simulink model "Lista3"  (R2023a)
settings: Solver=VariableStepAuto  StartTime=0.0  StopTime=10.0  RelTol=1e-3
libraries: fl_lib x5, nesl_utility x2
settings Model: Creator=gutoc  LastModifiedBy=gutoc

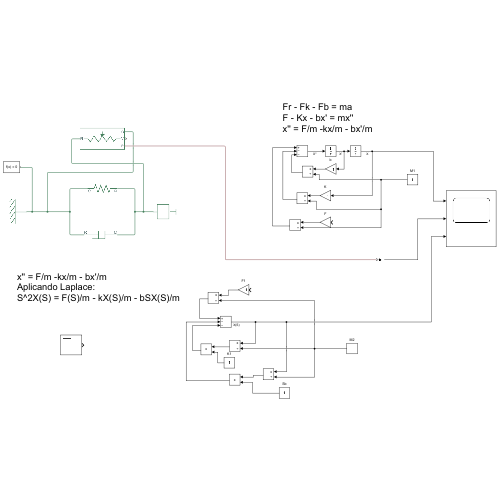
[thumbnail: Simulink's stored preview of the top-level diagram]
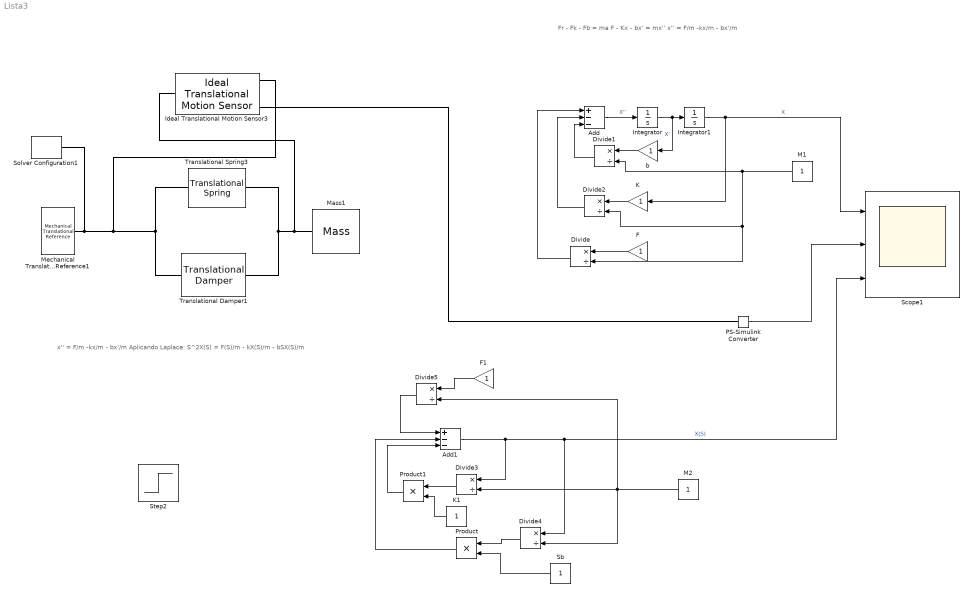
== system Lista3 ==
  note: x'' = F/m -kx/m - bx'/m
      | Aplicando Laplace:
      | S^2X(S) = F(S)/m - kX(S)/m - bSX(S)/m
  note: Fr - Fk - Fb = ma
      | F - Kx - bx' = mx''
      | x'' = F/m -kx/m - bx'/m
  Add : Sum  Inputs=+--
  Add1 : Sum  Inputs=+--
  Divide{,1..5} (6 alike) : Product  Inputs=*/
  F : Gain
  F1 : Gain
  Ideal Translational Motion Sensor3 : fl_lib/Mechanical/Mechanical Sensors/Ideal Translational Motion Sensor  reference=foundation.enum.MeasurementReference.difference  acceleration_port=false  velocity_port=true  position_port=true  offset=0 m
  Integrator : Integrator
  Integrator1 : Integrator
  K : Gain
  K1 : Constant
  M1 : Constant  VectorParams1D=off
  M2 : Constant  VectorParams1D=off
  Mass1 : fl_lib/Mechanical/Translational Elements/Mass  mass=10 kg  num_ports=foundation.enum.numPorts2.one  v_specify=on  v_priority=High  v=5 m/s  v_nominal_specify=off  v_nominal_unit=m/s  v_nominal_value=1  f_specify=off  f_priority=None  f=0 N  f_nominal_specify=off  f_nominal_unit=N  f_nominal_value=1
  Mechanical Translational Reference1 : fl_lib/Mechanical/Translational Elements/Mechanical Translational Reference
  PS-Simulink Converter : nesl_utility/PS-Simulink Converter  PhysicalDomain=network_engine_domain  SubClassName=ps_output  LeftPortType=input  RightPortType=output  PseudoPeriodic=off  Frequencies=[]  VectorFormat=inherit  Unit=inherit  AffineConversion=off
  Product : Product
  Product1 : Product
  Sb : Constant  VectorParams1D=off
  Scope1 : Scope  NumInputPorts=3
  Solver Configuration1 : nesl_utility/Solver Configuration  PhysicalDomain=network_engine_domain  SubClassName=solver  LeftPortType=input  RightPortType=generic  Tones=[]  Harmonics=[]  SimulateNoise=off  Profile=off  UseLocalSampling=off  EnableSwitchedLinearOptims=on  FrequencyDomain=off  UseCCode=off  RelTol=0.001  AbsTol=1e-06  MinStep=1e-09  ToWorkspace=off  RevertToSquareIcSolve=off  NumHomotopyIterations=100  PhasorMode=off  PhasorModeNumHarmonics=1  ConsistencySolver=NEWTON_FTOL  IndexReductionMethod=DerivativeReplacement  DoDC=off  ResidualTolerance=1e-09  ConsistencyTolSource=GLOBAL  ConsistencyAbsTol=0.001  ConsistencyRelTol=0.001  ConsistencyTolFactor=0.001  UseLocalSolver=off  LocalSolverChoice=NE_BACKWARD_EULER_ADVANCER  ResolveIndetEquations=on  FunctionEvalNumThread=1  LocalSolverSampleTime=0.001  DoFixedCost=off  MaxNonlinIter=3  MaxModeIter=2  ComputeImpulses=off  ImpulseIterations=2  LinearAlgebra=Sparse  LinearAlgebraNumThread=0  EquationFormulation=NE_TIME_EF  DelaysMemoryBudget=1024  AutomaticFiltering=on  FilteringTimeConstant=0.001  PartitionStorageMethod=AS_NEEDED  PartitionMemoryBudget=1024  PartitionMethod=FAST
  Step2 : Step  Before=10  SampleTime=0
  Translational Damper1 : fl_lib/Mechanical/Translational Elements/Translational Damper  D=100 N/(m/s)  v_specify=off  v_priority=None  v=0 m/s  v_nominal_specify=off  v_nominal_unit=m/s  v_nominal_value=1  f_specify=off  f_priority=None  f=0 N  f_nominal_specify=off  f_nominal_unit=N  f_nominal_value=1
  Translational Spring3 : fl_lib/Mechanical/Translational Elements/Translational Spring  spr_rate=1000 N/m  v_specify=off  v_priority=None  v=0 m/s  v_nominal_specify=off  v_nominal_unit=m/s  v_nominal_value=1  f_specify=off  f_priority=None  f=0 N  f_nominal_specify=off  f_nominal_unit=N  f_nominal_value=1  x_specify=off  x_priority=High  x=0 m  x_nominal_specify=off  x_nominal_unit=m  x_nominal_value=1
  b : Gain
  wires:
  Add/1 -> Integrator/1  "X''"
  Integrator/1 -> b/1, Integrator1/1  "X'"
  F/1 -> Divide/1
  Divide/1 -> Add/1
  b/1 -> Divide1/1
  Divide1/1 -> Add/3
  M1/1 -> Divide1/2, Divide2/2, Divide/2
  K/1 -> Divide2/1
  Divide2/1 -> Add/2
  Add1/1 -> Scope1/3, Divide4/1, Divide3/1  "X(S)"
  Divide4/1 -> Product/1
  Product/1 -> Add1/2
  Sb/1 -> Product/2
  Divide3/1 -> Product1/1
  Product1/1 -> Add1/3
  M2/1 -> Divide4/2, Divide5/2, Divide3/2
  Divide5/1 -> Add1/1
  F1/1 -> Divide5/1
  Integrator1/1 -> Scope1/1, K/1  "X"
  PS-Simulink Converter/1 -> Scope1/2
  K1/1 -> Product1/2
  connections:
  Translational Spring3/LConn1 -- Translational Damper1/RConn1 -- Ideal Translational Motion Sensor3/LConn1 -- Mass1/LConn1
  PS-Simulink Converter/LConn1 -- Ideal Translational Motion Sensor3/RConn3
  Translational Spring3/RConn1 -- Ideal Translational Motion Sensor3/RConn1 -- Solver Configuration1/RConn1 -- Mechanical Translational Reference1/LConn1 -- Translational Damper1/LConn1
